simulink model "pathPlanningBicycleSimulinkModelTest"  (R2022a)
settings: Solver=VariableStepAuto  StartTime=0.0  StopTime=10000  RelTol=1e-3
model workspace (MAT data in the model file):
  Sig = Simulink.Signal
  Sig.DataType = 'auto'
  Sig.Dimensions = -1
  Sig.DimensionsMode = 'auto'
  Sig.Complexity = 'auto'
  Sig.SampleTime = -1
  Sig.SamplingMode = 'auto'
values from neighbouring files (symbols this model uses):
  goalLoc = [0 0]    [Generate_Trajectory.m]    (also in Trajectory_Generate.m = [x(end),y(end)]; Trajectory_Generate_Circumference.m = [x(end),y(end)]; Trajectory_Generate_Line.m = [x(end),y(end)]; Trajectory_Generate_Straigth.m = [x(end),y(end)])
  startLoc = [0 0]    [Generate_Trajectory.m]    (also in Trajectory_Generate.m = [x(1),y(1)]; Trajectory_Generate_Circumference.m = [x(1),y(1)]; Trajectory_Generate_Line.m = [x(1),y(1)]; Trajectory_Generate_Straigth.m = [x(1),y(1)])
  Waypoints = [15 15;20 15]    [Generate_Trajectory.m]
libraries: robotmobilelib x2, robotalgslib x1
settings Model: Creator=The MathWorks, Inc.  LastModifiedBy=Gabriel-PC
settings SolverCC: AlgebraicLoopSolver=TrustRegion
settings DebuggingCC: UnconnectedInputMsg=warning  UnconnectedOutputMsg=warning  UnconnectedLineMsg=warning  SymbolicDimsDataTypeCodeGenerationDiagnostic=none  SFMachineParentedDataDiag=warning
settings RTWCC: DLArmComputeVersion=19.05

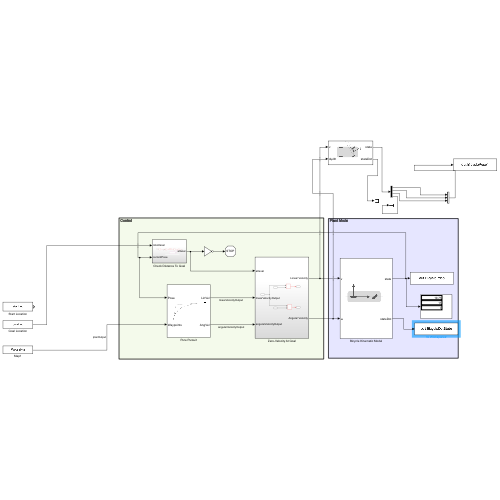
[thumbnail: Simulink's stored preview of the top-level diagram]
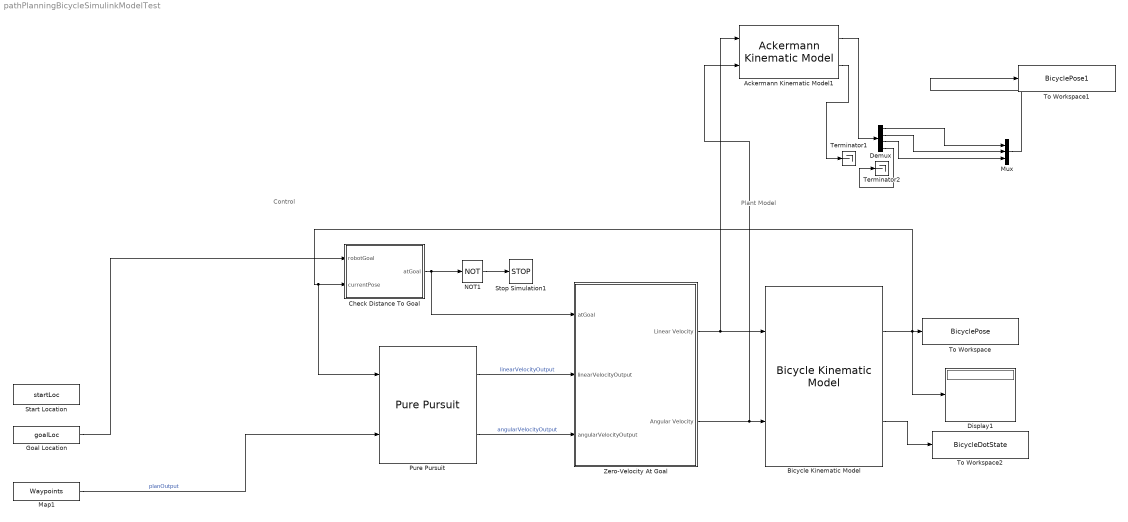
== system pathPlanningBicycleSimulinkModelTest ==
  note: Control
  note: Plant Model
  Ackermann Kinematic Model1 : robotmobilelib/Ackermann Kinematic Model  WheelBase=0.6  VehicleSpeedRange=[-inf inf]  MaxSteeringAngle=pi/4  InitialState=[5; 5; 0; 0]  SimulateUsing=Interpreted execution
      settings: SourceProductBaseCode=RO
  Bicycle Kinematic Model : robotmobilelib/Bicycle Kinematic Model  VehicleInputs=Vehicle Speed & Heading Angular Velocity  WheelBase=0.5  VehicleSpeedRange=[-inf, inf]  MaxSteeringAngle=pi/3  InitialState=[15; 15; 0]  SimulateUsing=Interpreted execution
      settings: SourceProductBaseCode=RO
  Check Distance To Goal : Subsystem
  Demux : Demux
  Display1 : Display
  Goal Location : Constant  Value=goalLoc
  Map1 : Constant  Value=Waypoints
  Mux : Mux  Inputs=3
  NOT1 : Logic  Operator=NOT  IconShape=distinctive  AllPortsSameDT=off  OutDataTypeStr=boolean
  Pure Pursuit : robotalgslib/Pure Pursuit  DesiredLinearVelocity=0.5  MaxAngularVelocity=1.0  LookaheadDistance=0.5  TargetDirPort=off  SimulateUsing=Code generation
  Start Location : Constant  Value=startLoc
  Stop Simulation1 : Stop
  Terminator1 : Terminator
  Terminator2 : Terminator
  To Workspace : ToWorkspace  VariableName=BicyclePose  SampleTime=-1
  To Workspace1 : ToWorkspace  VariableName=BicyclePose1  SampleTime=-1
  To Workspace2 : ToWorkspace  VariableName=BicycleDotState  SampleTime=-1
  Zero-Velocity At Goal : Subsystem
  wires:
  Goal Location/1 -> Check Distance To Goal/1(robotGoal)
  Check Distance To Goal/1(atGoal) -> Zero-Velocity At Goal/1(atGoal), NOT1/1
  Zero-Velocity At Goal/2(Angular Velocity) -> Ackermann Kinematic Model1/2, Bicycle Kinematic Model/2
  NOT1/1 -> Stop Simulation1/1
  Pure Pursuit/1 -> Zero-Velocity At Goal/2(linearVelocityOutput)  "linearVelocityOutput"
  Bicycle Kinematic Model/2 -> To Workspace2/1
  Pure Pursuit/2 -> Zero-Velocity At Goal/3(angularVelocityOutput)  "angularVelocityOutput"
  Zero-Velocity At Goal/1(Linear Velocity) -> Ackermann Kinematic Model1/1, Bicycle Kinematic Model/1
  Ackermann Kinematic Model1/1 -> Demux/1
  Demux/1 -> Mux/1
  Demux/2 -> Mux/2
  Demux/3 -> Mux/3
  Mux/1 -> To Workspace1/1
  Ackermann Kinematic Model1/2 -> Terminator1/1
  Demux/4 -> Terminator2/1
  Bicycle Kinematic Model/1 -> Pure Pursuit/1, Check Distance To Goal/2(currentPose), Display1/1, To Workspace/1
  Map1/1 -> Pure Pursuit/2  "planOutput"

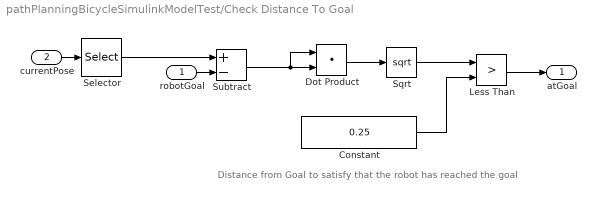
== system pathPlanningBicycleSimulinkModelTest/Check Distance To Goal ==
  note: Distance from Goal to satisfy that the robot has reached the goal
  robotGoal : Inport
  currentPose : Inport  Port=2
  Constant : Constant  Value=0.25
  Dot Product : DotProduct  OutDataTypeStr=Inherit: Inherit via internal rule
  Less Than : RelationalOperator  Operator=>  OutDataTypeStr=boolean  RndMeth=Simplest  InputSameDT=off
  Selector : Selector  InputPortWidth=3  IndexOptions=Index vector (dialog)  Indices=[1 2]  OutputSizes=1
  Sqrt : Sqrt
  Subtract : Sum  Inputs=+-
  atGoal : Outport
  wires:
  robotGoal/1 -> Subtract/2
  Dot Product/1 -> Sqrt/1
  Constant/1 -> Less Than/2
  currentPose/1 -> Selector/1
  Less Than/1 -> atGoal/1
  Sqrt/1 -> Less Than/1
  Subtract/1 -> Dot Product/1, Dot Product/2
  Selector/1 -> Subtract/1

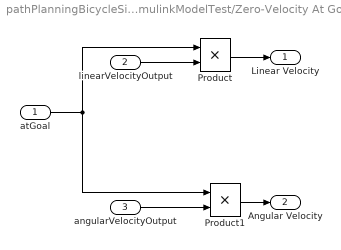
== system pathPlanningBicycleSimulinkModelTest/Zero-Velocity At Goal ==
  atGoal : Inport
  linearVelocityOutput : Inport  Port=2
  angularVelocityOutput : Inport  Port=3
  Product : Product
  Product1 : Product
  Linear Velocity : Outport  OutDataTypeStr=double
  Angular Velocity : Outport  Port=2  OutDataTypeStr=double
  wires:
  atGoal/1 -> Product1/1, Product/1
  angularVelocityOutput/1 -> Product1/2
  linearVelocityOutput/1 -> Product/2
  Product/1 -> Linear Velocity/1
  Product1/1 -> Angular Velocity/1
